simulink subsystem "Magnetometer_MMC5983MA"  (R2025b)
settings: Solver=VariableStepAuto  StartTime=0.0  StopTime=10.0  RelTol=1e-3
settings Model: Creator=slee7  LastModifiedBy=slee7

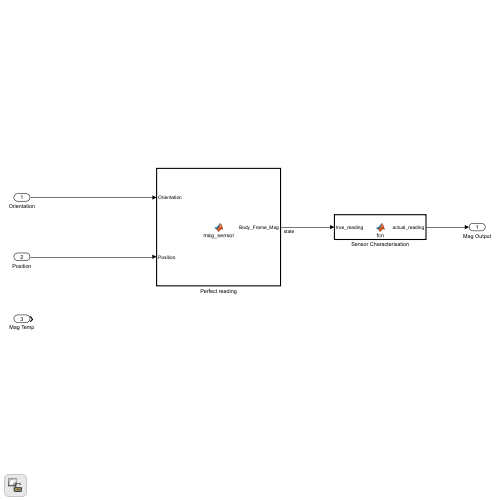
[thumbnail: Simulink's stored preview of the top-level diagram]
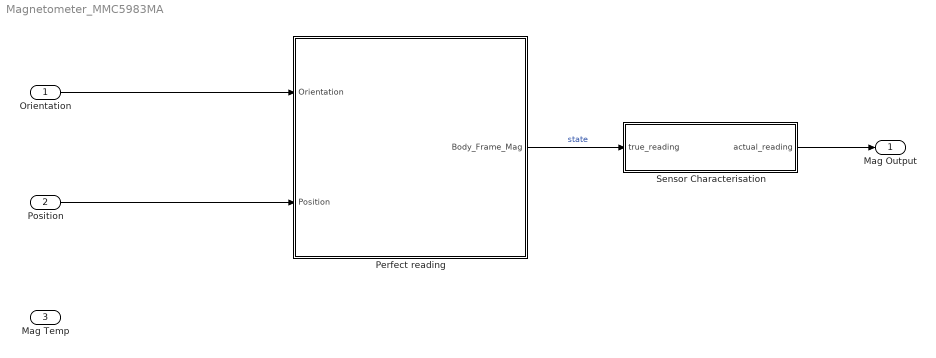
== system Magnetometer_MMC5983MA ==
  Orientation : Inport
  Position : Inport  Port=2
  Mag Temp : Inport  Port=3
  Perfect reading : MATLAB Function  TreatAsAtomicUnit=on
  Sensor Characterisation : MATLAB Function  TreatAsAtomicUnit=on
  Mag Output : Outport
  wires:
  Sensor Characterisation/1(actual_reading) -> Mag Output/1
  Perfect reading/1(Body_Frame_Mag) -> Sensor Characterisation/1(true_reading)  "state"
  Orientation/1 -> Perfect reading/1(Orientation)
  Position/1 -> Perfect reading/2(Position)

== matlab function Magnetometer_MMC5983MA/Sensor Characterisation ==
  data: true_reading input; actual_reading output
function actual_reading = fcn(true_reading)
    persistent b_previous

    % Spherical Calibration
   
    b = [-0.0705; -0.1152; 0.0250];
    A = [2.2439, -0.0154, -0.0144;
        -0.0154, 2.2042, -0.097;
        -0.0144, -0.0097, 2.4001];

    % Hard-Iron Bias (Offset)
    cal_reading = true_reading - b;

    % Soft-Iron Bias (Scale Distortion)
    cal_reading = A * cal_reading;


    dt = 0.02; % CAN Bus limit 20 ms
    % Simulation Time Step for BW=11 (Measurement Time): 0.0005

    % Bias: Composite Bias = Const + Gauss-Markov Drift
    
        b_const = [0; 0; 0]; % Constant bias
    
        % Drift bias b_{k+1} &= e^{-\Delta t/ \tau} * b_k + \omega_k
        
        if isempty(b_previous)
            b_previous = [0; 0; 0]; 
        end
    
        tau = [6.9630; 7.8914; 6.3777]; % time constant of drift
        q = [1.1384e-11; 2.9369e-11; 4.0735e-11]; % variance on drift
    
        omega = sqrt(q) .* randn(3,1); % omega ~ N(0,q)
        
        phi = exp(-dt ./ tau);
        b_drift = phi .* b_previous + omega;

        b_previous = b_drift;
    
        composite_bias = b_const + b_drift; 

    % Noise: Gaussian

        noise_std = [1.2; 1.2; 1.2];      % [Total RMS Noise for BW=11]
    
        noise = noise_std .* randn(3,1); % noise ~ N(0,noise_variance)
    
    % Quantisation:

        quant_step = [0.0625; 0.0625; 0.0625]; % Quant Step (for 18-bit)
   

    % Reading Processing:

        actual_reading_continuous  = cal_reading(:) + composite_bias + noise;

        actual_reading_quantised = quant_step * round(actual_reading_continuous/quant_step);

        actual_reading = actual_reading_quantised;

end

% Currently Ignoring: 
% Scale_factor_error 
% Misalignment_error

== matlab function Magnetometer_MMC5983MA/Perfect reading ==
  data: Body_Frame_Mag output; Orientation input; Position input
function Body_Frame_Mag = mag_sensor(Orientation, Position)
%#codegen

height = Position(2) % Altitude in meters
lat = 51.49897; % Latitude
lon = -0.17430; % Longitude
time = decyear(2025,2,24); % Convert date to decimal year

% Calculate Magnetic Field (WMM2025)
% XYZ = North, East, Down components (nT)
% H = Horizontal intensity
% DEC = Declination
% DIP = Inclination
% F = Total intensity
[B_w, H, DEC, DIP, F] = wrldmagm(height, lat, lon, time, '2025');

% Ensure column vectors
Orientation = Orientation(:);
B_w = B_w(:);

% Convert from nT to mG
B_w = B_w .* 100;

% Normalize quaternion
q = Orientation / norm(Orientation);

% Quaternion inverse (for unit quaternion)
q_inv = [q(1); -q(2:4)];

% Convert vector to pure quaternion
B_quat = [0; B_w];

% Perform rotation: B_b = q^{-1} * B_w * q, converting Earth magnetic field in NED frame to body frame
B_rot = quatmultiply(quatmultiply(q_inv.', B_quat.'), q.'); 

% Extract vector part
B_b = B_rot(2:4).';

end
